simulink model "Nyquist"  (R2022a)
settings: Solver=VariableStepAuto  StartTime=0.0  StopTime=100  RelTol=1e-3
libraries: simulink_extras x6
settings Model: Creator=anthony  LastModifiedBy=anthony

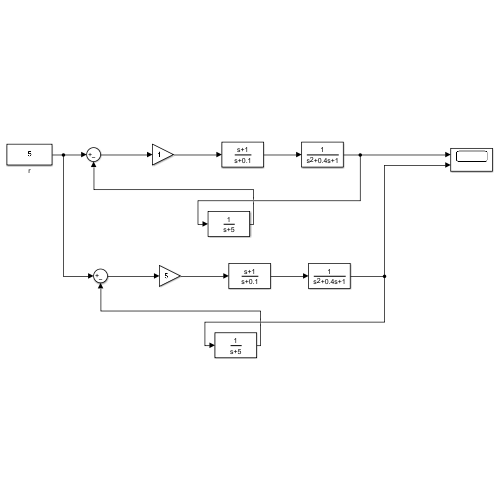
[thumbnail: Simulink's stored preview of the top-level diagram]
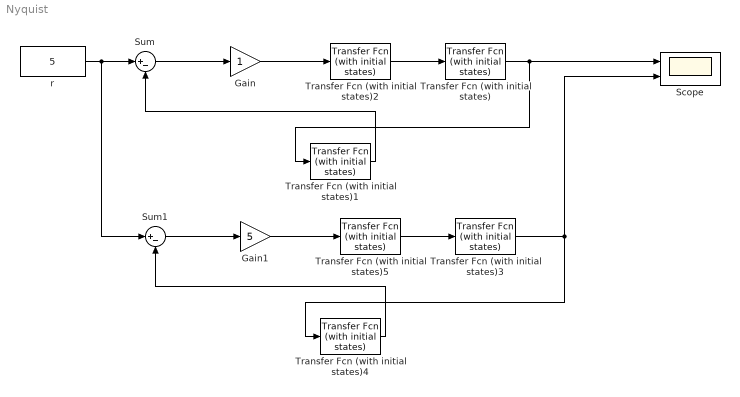
== system Nyquist ==
  Gain : Gain
  Gain1 : Gain  Gain=5
  Scope : Scope  NumInputPorts=2
  Sum : Sum  Inputs=|+-
  Sum1 : Sum  Inputs=|+-
  Transfer Fcn (with initial states) : simulink_extras/Additional Linear/Transfer Fcn (with initial states)  N=[1]  D=[1 0.4 1]  X0=0
  Transfer Fcn (with initial states)1 : simulink_extras/Additional Linear/Transfer Fcn (with initial states)  N=[1]  D=[1 5]  X0=0
  Transfer Fcn (with initial states)2 : simulink_extras/Additional Linear/Transfer Fcn (with initial states)  N=[1 1]  D=[1 0.1]  X0=0
  Transfer Fcn (with initial states)3 : simulink_extras/Additional Linear/Transfer Fcn (with initial states)  N=[1]  D=[1 0.4 1]  X0=0
  Transfer Fcn (with initial states)4 : simulink_extras/Additional Linear/Transfer Fcn (with initial states)  N=[1]  D=[1 5]  X0=0
  Transfer Fcn (with initial states)5 : simulink_extras/Additional Linear/Transfer Fcn (with initial states)  N=[1 1]  D=[1 0.1]  X0=0
  r : Constant  Value=5
  wires:
  Sum/1 -> Gain/1
  Gain/1 -> Transfer Fcn (with initial states)2/1
  Transfer Fcn (with initial states)2/1 -> Transfer Fcn (with initial states)/1
  Transfer Fcn (with initial states)/1 -> Scope/1, Transfer Fcn (with initial states)1/1
  Transfer Fcn (with initial states)1/1 -> Sum/2
  Transfer Fcn (with initial states)4/1 -> Sum1/2
  Transfer Fcn (with initial states)3/1 -> Scope/2, Transfer Fcn (with initial states)4/1
  Transfer Fcn (with initial states)5/1 -> Transfer Fcn (with initial states)3/1
  r/1 -> Sum1/1, Sum/1
  Gain1/1 -> Transfer Fcn (with initial states)5/1
  Sum1/1 -> Gain1/1
